simulink model "Roberto Graham's work"  (R2023b)
settings: Solver=VariableStepAuto  StartTime=0.0  StopTime=10.0  RelTol=1e-3
undefined symbols (not defined in the file or in its folder): carData
settings Model: Creator=robertgraham  LastModifiedBy=robertgraham

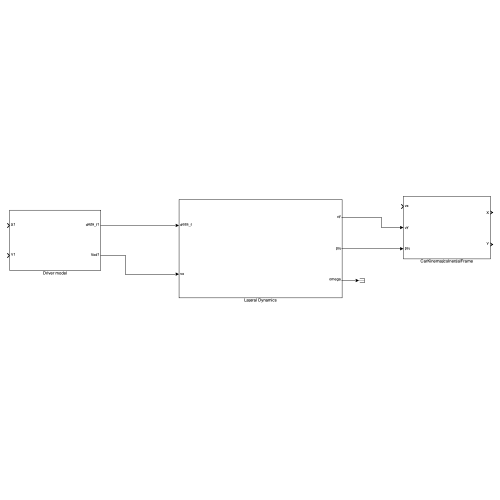
[thumbnail: Simulink's stored preview of the top-level diagram]
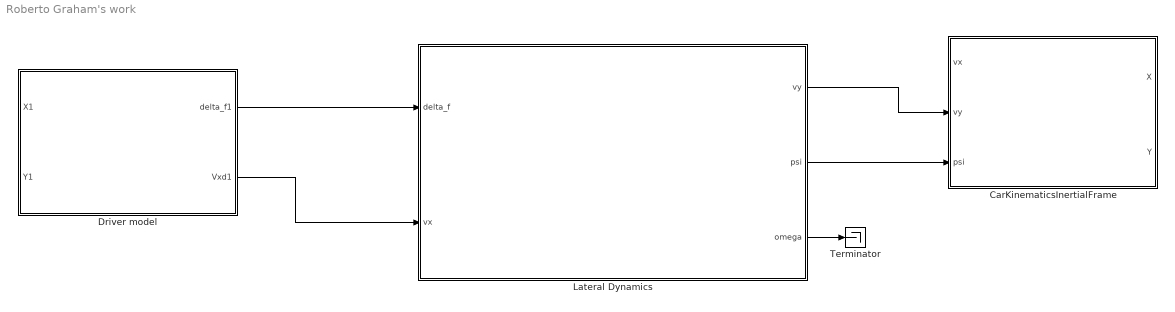
== system Roberto Graham's work ==
  CarKinematicsInertialFrame : Subsystem
  Driver model : Subsystem
  Lateral Dynamics : Subsystem
  Terminator : Terminator
  wires:
  Driver model/1(delta_f1) -> Lateral Dynamics/1(delta_f)
  Driver model/2(Vxd1) -> Lateral Dynamics/2(vx)
  Lateral Dynamics/1(vy) -> CarKinematicsInertialFrame/2(vy)
  Lateral Dynamics/2(psi) -> CarKinematicsInertialFrame/3(psi)
  Lateral Dynamics/3(omega) -> Terminator/1

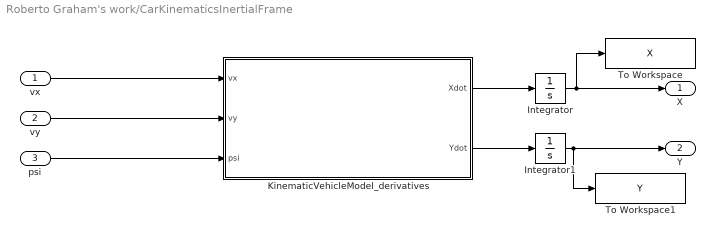
== system Roberto Graham's work/CarKinematicsInertialFrame ==
  vx : Inport
  vy : Inport  Port=2
  psi : Inport  Port=3
  Integrator : Integrator  InitialCondition=carData.init.X0
  Integrator1 : Integrator  InitialCondition=carData.init.Y0
  KinematicVehicleModel_derivatives : MATLAB Function  TreatAsAtomicUnit=on  mask{obj=carData}
      mask prompts: obj "obj structure"
  To Workspace : ToWorkspace  VariableName=X  SaveFormat=Timeseries  SampleTime=-1
  To Workspace1 : ToWorkspace  VariableName=Y  SaveFormat=Timeseries  SampleTime=-1
  X : Outport
  Y : Outport  Port=2
  wires:
  KinematicVehicleModel_derivatives/1(Xdot) -> Integrator/1
  KinematicVehicleModel_derivatives/2(Ydot) -> Integrator1/1
  Integrator/1 -> To Workspace/1, X/1
  Integrator1/1 -> To Workspace1/1, Y/1
  vx/1 -> KinematicVehicleModel_derivatives/1(vx)
  vy/1 -> KinematicVehicleModel_derivatives/2(vy)
  psi/1 -> KinematicVehicleModel_derivatives/3(psi)

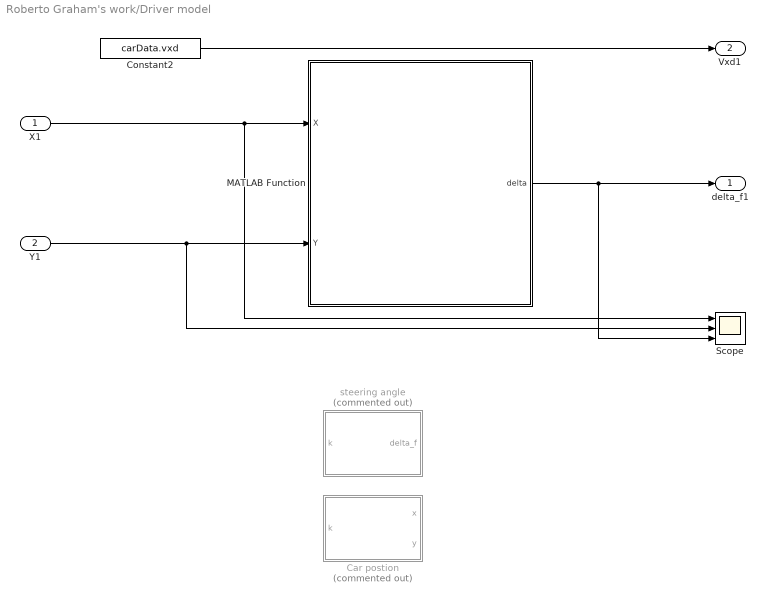
== system Roberto Graham's work/Driver model ==
  X1 : Inport
  Y1 : Inport  Port=2
  "Car postion " : MATLAB Function  Commented=on  TreatAsAtomicUnit=on
  Constant2 : Constant  Value=carData.vxd
  MATLAB Function : MATLAB Function  TreatAsAtomicUnit=on
  Scope : Scope  NumInputPorts=3
  steering angle : MATLAB Function  Commented=on  TreatAsAtomicUnit=on
  delta_f1 : Outport
  Vxd1 : Outport  Port=2
  wires:
  MATLAB Function/1(delta) -> delta_f1/1, Scope/3
  Constant2/1 -> Vxd1/1
  X1/1 -> Scope/1, MATLAB Function/1(X)
  Y1/1 -> Scope/2, MATLAB Function/2(Y)

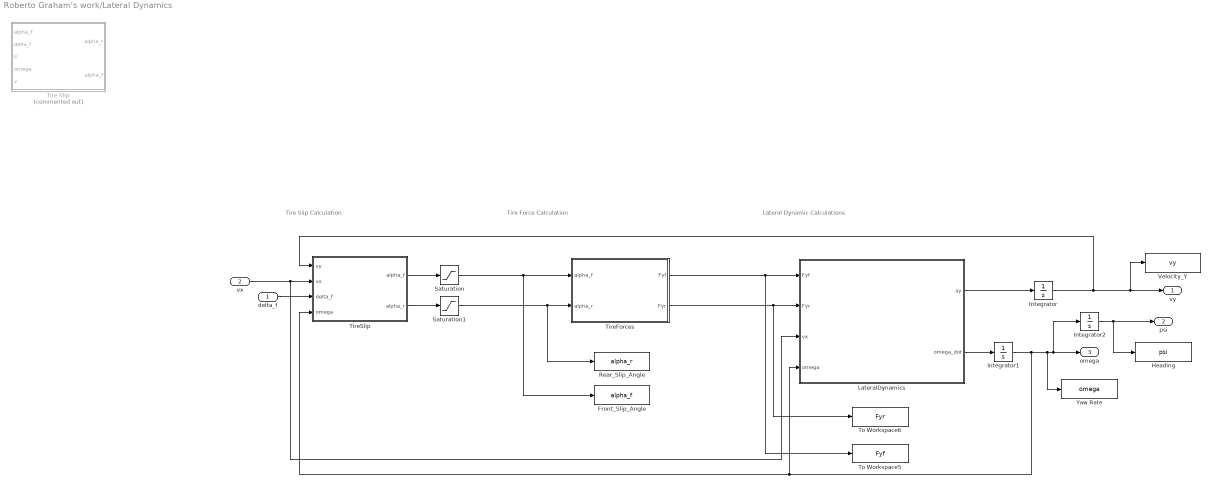
== system Roberto Graham's work/Lateral Dynamics ==
  note: Tire Force Calculation
  note: Tire Slip Calculation
  note: Lateral Dynamic Calculations
  delta_f : Inport
  vx : Inport  Port=2
  " Tire Slip" : MATLAB Function  Commented=on  TreatAsAtomicUnit=on
  Front_Slip_Angle : ToWorkspace  VariableName=alpha_f  SaveFormat=Timeseries  SampleTime=-1
  Heading : ToWorkspace  VariableName=psi  SaveFormat=Timeseries  SampleTime=-1
  Integrator : Integrator  InitialCondition=carData.init.vy0
  Integrator1 : Integrator  InitialCondition=carData.init.omega0
  Integrator2 : Integrator  InitialCondition=carData.init.psi0
  LateralDynamics : MATLAB Function  TreatAsAtomicUnit=on  mask{obj=carData}
      mask prompts: obj "obj structure"
  Rear_Slip_Angle : ToWorkspace  VariableName=alpha_r  SaveFormat=Timeseries  SampleTime=-1
  Saturation : Saturate  UpperLimit=carData.maxAlpha  LowerLimit=-carData.maxAlpha
  Saturation1 : Saturate  UpperLimit=carData.maxAlpha  LowerLimit=-carData.maxAlpha
  TireForces : MATLAB Function  TreatAsAtomicUnit=on  mask{obj=carData}
      mask prompts: obj "obj structure"
  TireSlip : MATLAB Function  TreatAsAtomicUnit=on  mask{obj=carData}
      mask prompts: obj "obj structure"
  To Workspace5 : ToWorkspace  VariableName=Fyf  SaveFormat=Timeseries  SampleTime=-1
  To Workspace6 : ToWorkspace  VariableName=Fyr  SaveFormat=Timeseries  SampleTime=-1
  Velocity_Y : ToWorkspace  VariableName=vy  SaveFormat=Timeseries  SampleTime=-1
  Yaw Rate : ToWorkspace  VariableName=omega  SaveFormat=Timeseries  SampleTime=-1
  vy : Outport
  psi : Outport  Port=2
  omega : Outport  Port=3
  wires:
  TireSlip/2(alpha_r) -> Saturation1/1
  Saturation1/1 -> TireForces/2(alpha_r), Rear_Slip_Angle/1
  Integrator1/1 -> Integrator2/1, omega/1, Yaw Rate/1, LateralDynamics/4(omega), TireSlip/4(omega)
  Integrator/1 -> vy/1, Velocity_Y/1, TireSlip/1(vy)
  Integrator2/1 -> Heading/1, psi/1
  LateralDynamics/1(ay) -> Integrator/1
  Saturation/1 -> TireForces/1(alpha_f), Front_Slip_Angle/1
  TireForces/2(Fyr) -> LateralDynamics/2(Fyr), To Workspace6/1
  vx/1 -> TireSlip/2(vx), LateralDynamics/3(vx)
  delta_f/1 -> TireSlip/3(delta_f)
  TireSlip/1(alpha_f) -> Saturation/1
  LateralDynamics/2(omega_dot) -> Integrator1/1
  TireForces/1(Fyf) -> LateralDynamics/1(Fyf), To Workspace5/1

== matlab function Roberto Graham's work/Driver model/Car postion  ==
  data: k input; x output; y output
function [x,y] = fcn(k)

% find delta_f steering angle
% input should be X and Y value

x = xc(k);
y = yc(k);

== matlab function Roberto Graham's work/Driver model/steering angle ==
  data: k input; delta_f output
function delta_f = fcn(k)

% find delta_f steering angle
% input should be X and Y value

delta_f = atan2(yc(k)-yp(k),xc(k)- xp(k));

== matlab function Roberto Graham's work/Lateral Dynamics/ Tire Slip ==
  data: alpha_f input; delta_f input; alpha_r output; lr input; omega input; v input; alpha_f output
function [alpha_r,alpha_f] = fcn(alpha_f,delta_f,lr,omega,v)


alpha_r = atan2(vy-lr*omega,vx);

alpha_f = delta_f - atan2(vy+lf*omega,vx);

== matlab function Roberto Graham's work/Lateral Dynamics/LateralDynamics ==
  data: Fyf input; Fyr input size=1; vx input; omega input; ay output; obj parameter; omega_dot output
function [ay, omega_dot] = fcn(Fyf, Fyr, vx, omega, obj)

Fy = Fyf + Fyr;
ay = Fy / obj.Mass - omega * vx;
        
M  = Fyf * obj.lf - Fyr * obj.lr;        
omega_dot = M / obj.Inertia;        

end

== matlab function Roberto Graham's work/CarKinematicsInertialFrame/KinematicVehicleModel_derivatives ==
  data: vx input; vy input; psi input size=1; Xdot output; Ydot output
function [Xdot, Ydot] = fcn(vx, vy, psi)
    temp = TF(psi) * [vx;vy]; 
    Xdot = temp(1);
    Ydot = temp(2);
  
end

function y = TF(psi)
    y = [cos(psi), -sin(psi); sin(psi), cos(psi)];
end

== matlab function Roberto Graham's work/Lateral Dynamics/TireSlip ==
  data: vy input size=1; vx input; delta_f input size=1; omega input; alpha_f output; obj parameter; alpha_r output
function [alpha_f, alpha_r] = fcn(vy,  vx, delta_f, omega, obj)


if abs(vx)> obj.vx_threshold1
      alpha_r = atan2(vy-lr*omega,vx);
      alpha_f = delta_f - atan2(vy+lf*omega,vx);
else
      alpha_f = 0;
      alpha_r = 0;
end



end

== matlab function Roberto Graham's work/Lateral Dynamics/TireForces ==
  data: alpha_f input; alpha_r input; Fyf output; obj parameter; Fyr output
function [Fyf, Fyr] = fcn(alpha_f, alpha_r, obj)

Fyf = min(obj.Fyfmax,obj.Calpha_f * alpha_f);
Fyr = min(obj.Fyrmax, obj.Calpha_r * alpha_r);
end

== matlab function Roberto Graham's work/Driver model/MATLAB Function ==
  data: X input; delta output; Y input
function delta = SimplestDriver(X,Y)

%===============================
if abs(Y)<0.5
    delta = 0;
elseif abs(Y - 400) < 0.5
    delta = 0;
elseif X > 900
    delta = 5;
else
    delta = -5;
end



%===============================
% if X > 900
%     delta = 5;
% elseif X < 0
%     delta = -5;
% else
%     delta = 0;
% end

%===============================
% if X > 900
%     delta = 5;
% elseif X < 0
%     delta = 5;
% else
%     delta = 0;
% end
